simulink model "testAntennaVsArray"  (R2025b)
settings: Solver=VariableStepAuto  StartTime=0.0  StopTime=0.01  RelTol=1e-3
libraries: dspstat3 x4, rfmathmodels2 x2, phasedwavlib x1
settings Model: Creator=galberti  LastModifiedBy=galberti

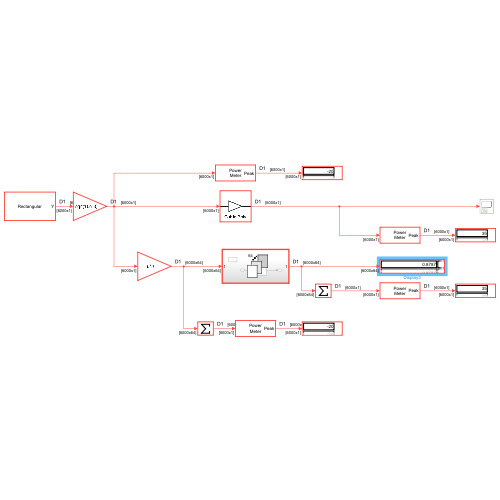
[thumbnail: Simulink's stored preview of the top-level diagram]
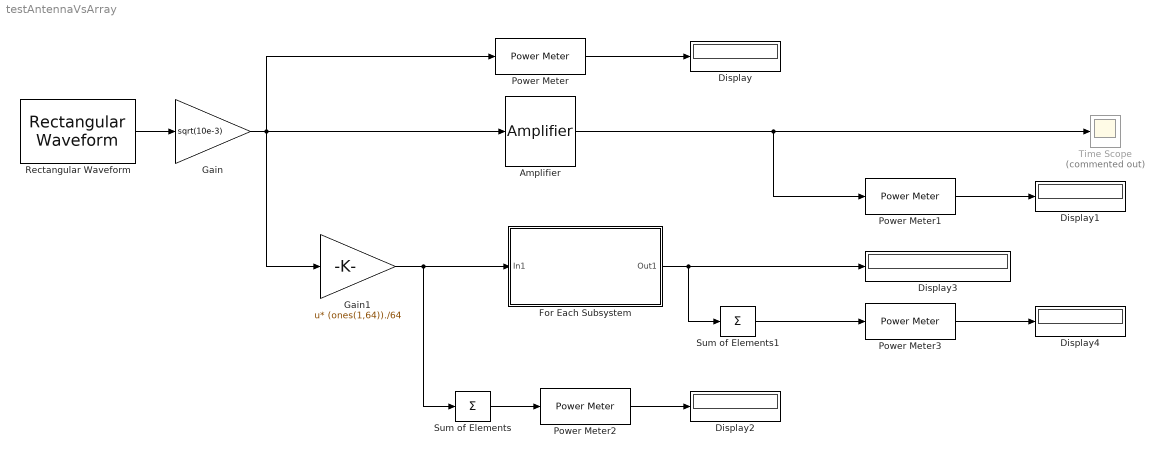
== system testAntennaVsArray ==
  Amplifier : rfmathmodels2/Amplifier  Model=cubic  Gain=55  Nonlinearity=OIP3  IIP3=Inf  OIP3=Inf  IP1dB=Inf  OP1dB=Inf  IPsat=Inf  OPsat=Inf  Table=[ -25, 5, -1; -10, 20, -2; 0, 27, 5; 5, 28, 12 ]  MagnitudeGainDB=0  Vsat=1  MagnitudeSmooth=2  PhaseGainRadian=-.45  PhaseSaturation=.88  PhaseSmooth=[ 3.43, 3.43 ]  InputScaleDB=0  AmAmParameters=[ 2.1587, 1.1517 ]  AmPmParameters=[ 4.0033, 9.1040 ]  OutputScaleDB=0  SimulateUsing=Interpreted execution  IncludeNoise=off  NoiseType=NF  NoiseTemperature=290  NF=10 * log10( 2 )  NoiseFactor=2  SeedSource=auto  Seed=67987  SampleRate=1e6
  Display{,1..4} (5 alike) : Display
  For Each Subsystem : Subsystem  TreatAsAtomicUnit=on
  Gain : Gain  Gain=sqrt(10e-3)
  Gain1 : Gain  Gain=(ones(1,64))./64  Multiplication=Matrix(u*K)
  Power Meter{,1..3} (4 alike) : dspstat3/Power Meter  Measurement=Peak power  ReferenceLoad=1  OutputPowerUnits=dBW  WindowLength=256  OverlapLength=255  AllowArbitraryInputLength=off  ComputeCCDF=off  PowerRange=50  PowerResolution=0.1  CCDFOutput=Relative power (dB above average power)  ProbabilityVector=[ 10; 1; 0.1; 0.01; 0.001; 0.0001 ]  RelativePowerVector=[ 0; 3; 6; 9; 12 ]  ResetPort=off  SimulateUsing=Interpreted execution
  Rectangular Waveform : phasedwavlib/Rectangular Waveform  SampleRate=3e6  DurationSpecification=Pulse width  PulseWidth=1e-6  DutyCycle=0.5  PRF=500  PRFSelectionInputPort=off  SimulationTimeSource=Derive from waveform parameters  FrequencyOffsetSource=Property  FrequencyOffset=0  OutputFormat=Pulses  NumSamples=100  NumPulses=1  PRFOutputPort=off  CoefficientsOutputPort=off  SimulateUsing=Interpreted execution
  Sum of Elements : Sum  Inputs=+  CollapseMode=Specified dimension  CollapseDim=2
  Sum of Elements1 : Sum  Inputs=+  CollapseMode=Specified dimension  CollapseDim=2
  Time Scope : Scope  Commented=on
      settings: TimeUnits=Metric (based on Time Span)  ActiveDisplayYMinimum=-7.0292665648793617  ActiveDisplayYMaximum=63.263399083914273  YLabel=Amplitude
  wires:
  Rectangular Waveform/1 -> Gain/1
  Power Meter/1 -> Display/1
  Gain/1 -> Gain1/1, Amplifier/1, Power Meter/1
  Amplifier/1 -> Power Meter1/1, Time Scope/1
  Power Meter1/1 -> Display1/1
  Gain1/1 -> For Each Subsystem/1(In1), Sum of Elements/1
  Power Meter2/1 -> Display2/1
  Sum of Elements/1 -> Power Meter2/1
  For Each Subsystem/1(Out1) -> Display3/1, Sum of Elements1/1
  Sum of Elements1/1 -> Power Meter3/1
  Power Meter3/1 -> Display4/1

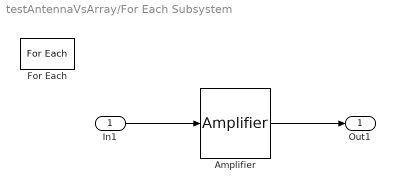
== system testAntennaVsArray/For Each Subsystem ==
  In1 : Inport  Partition=on  PartitionDimension=2  PartitionWidth=1  PartitionOffset=0
  Amplifier : rfmathmodels2/Amplifier  Model=cubic  Gain=55  Nonlinearity=OIP3  IIP3=Inf  OIP3=Inf  IP1dB=Inf  OP1dB=Inf  IPsat=Inf  OPsat=Inf  Table=[ -25, 5, -1; -10, 20, -2; 0, 27, 5; 5, 28, 12 ]  MagnitudeGainDB=0  Vsat=1  MagnitudeSmooth=2  PhaseGainRadian=-.45  PhaseSaturation=.88  PhaseSmooth=[ 3.43, 3.43 ]  InputScaleDB=0  AmAmParameters=[ 2.1587, 1.1517 ]  AmPmParameters=[ 4.0033, 9.1040 ]  OutputScaleDB=0  SimulateUsing=Interpreted execution  IncludeNoise=off  NoiseType=NF  NoiseTemperature=290  NF=10 * log10( 2 )  NoiseFactor=2  SeedSource=auto  Seed=67987  SampleRate=1e6
  For Each : ForEach  DisableCoverage=on
  Out1 : Outport  ConcatenationDimension=2
  wires:
  In1/1 -> Amplifier/1
  Amplifier/1 -> Out1/1
